simulink model "EZE557StEnCtrl"  (R2018b)
settings: Solver=FixedStepDiscrete  StartTime=0.0  StopTime=10.0  FixedStep=0.01  RelTol=1e-3
undefined symbols (not defined in the file or in its folder): data, KeSMSw4SSecRwLtStLgrstOtwdInwdClosePos1_Val, KeSMSw4SSecRwLtStLgrstUpwdDnwdClosePos1_Val, KeSMSw4SSecRwLtStLgrstUpwdDnwdClosePos2_Val, PassStBkReclnEn_Clear, PassStBkReclnEn_Set, PassStFwdBkwdEn_Clear, PassStFwdBkwdEn_Set, SecRwLtStBkReclnEn_Clear, SecRwLtStBkReclnEn_Set, SecRwLtStFwdBkwdEn_Clear, SecRwLtStFwdBkwdEn_Set, SecRwLtStLgrstInwdOtwdEn_Clear, SecRwLtStLgrstInwdOtwdEn_Set, SecRwLtStLgrstUpwdDnwdEn_Clear, SecRwLtStLgrstUpwdDnwdEn_Set, SecRwRtStBkReclnEn_Clear, SecRwRtStBkReclnEn_Set, SecRwRtStFwdBkwdEn_Clear, SecRwRtStFwdBkwdEn_Set, SecRwRtStLgrstInwdOtwdEn_Clear, SecRwRtStLgrstInwdOtwdEn_Set, SecRwRtStLgrstUpwdDnwdEn_Clear, SecRwRtStLgrstUpwdDnwdEn_Set, ThdRwLtStBkReclnEn_Clear, ThdRwLtStBkReclnEn_Set, ThdRwLtStCshnFldEn_Clear, ThdRwLtStCshnFldEn_Set, ThdRwLtStFwdBkwdEn_Clear, ThdRwLtStFwdBkwdEn_Set, ThdRwRtStBkReclnEn_Clear, ThdRwRtStBkReclnEn_Set, ThdRwRtStCshnFldEn_Clear, ThdRwRtStCshnFldEn_Set, ThdRwRtStFwdBkwdEn_Clear, ThdRwRtStFwdBkwdEn_Set, ZeroLEn_Clear, ZeroLEn_Set, ZeroREn_Clear, ZeroREn_Set
libraries: simulink x1
(part 2 of 2)

== system EZE557StEnCtrl/EZE557StEnCtrl_Cal_sys/Subsystem/If Action Subsystem24 ==
  Action Port : ActionPort
  Constant : Constant  Value=0  OutDataTypeStr=uint8
  ZeroREn_Set : FunctionCaller  FunctionPrototype=ZeroREn_Set(data)  InputArgumentSpecifications=uint8(1)  OutputArgumentSpecifications=<Enter example>
  wires:
  Constant/1 -> ZeroREn_Set/1

== system EZE557StEnCtrl/EZE557StEnCtrl_Cal_sys/Subsystem/If Action Subsystem25 ==
  note: Delete block
  Action Port : ActionPort
  Constant : Constant  Value=0  OutDataTypeStr=uint8
  SecRwLtStBkReclnEn_Set : FunctionCaller  FunctionPrototype=SecRwLtStBkReclnEn_Set(data)  InputArgumentSpecifications=uint8(1)  OutputArgumentSpecifications=<Enter example>
  wires:
  Constant/1 -> SecRwLtStBkReclnEn_Set/1

== system EZE557StEnCtrl/EZE557StEnCtrl_Cal_sys/Subsystem/If Action Subsystem26 ==
  note: Delete block
  Action Port : ActionPort
  Constant : Constant  Value=0  OutDataTypeStr=uint8
  SecRwRtStBkReclnEn_Set : FunctionCaller  FunctionPrototype=SecRwRtStBkReclnEn_Set(data)  InputArgumentSpecifications=uint8(1)  OutputArgumentSpecifications=<Enter example>
  wires:
  Constant/1 -> SecRwRtStBkReclnEn_Set/1

== system EZE557StEnCtrl/EZE557StEnCtrl_Cal_sys/Subsystem/If Action Subsystem27 ==
  note: Delete block
  Action Port : ActionPort
  Constant : Constant  Value=0  OutDataTypeStr=uint8
  PassStBkReclnEn_Clear : FunctionCaller  FunctionPrototype=PassStBkReclnEn_Clear(data)  InputArgumentSpecifications=uint8(1)
  wires:
  Constant/1 -> PassStBkReclnEn_Clear/1

== system EZE557StEnCtrl/EZE557StEnCtrl_Cal_sys/Subsystem/If Action Subsystem28 ==
  note: Delete block
  Action Port : ActionPort
  Constant : Constant  Value=0  OutDataTypeStr=uint8
  PassStBkReclnEn_Set : FunctionCaller  FunctionPrototype=PassStBkReclnEn_Set(data)  InputArgumentSpecifications=uint8(1)
  wires:
  Constant/1 -> PassStBkReclnEn_Set/1

== system EZE557StEnCtrl/EZE557StEnCtrl_Cal_sys/Subsystem/If Action Subsystem3 ==
  Action Port : ActionPort
  Constant : Constant  Value=0  OutDataTypeStr=uint8
  ThdRwLtStCshnFldEn_Set : FunctionCaller  FunctionPrototype=ThdRwLtStCshnFldEn_Set(data)  InputArgumentSpecifications=uint8(1)  OutputArgumentSpecifications=<Enter example>
  wires:
  Constant/1 -> ThdRwLtStCshnFldEn_Set/1

== system EZE557StEnCtrl/EZE557StEnCtrl_Cal_sys/Subsystem/If Action Subsystem4 ==
  Action Port : ActionPort
  Constant : Constant  Value=0  OutDataTypeStr=uint8
  ThdRwLtStCshnFldEn_Clear : FunctionCaller  FunctionPrototype=ThdRwLtStCshnFldEn_Clear(data)  InputArgumentSpecifications=uint8(1)  OutputArgumentSpecifications=<Enter example>
  wires:
  Constant/1 -> ThdRwLtStCshnFldEn_Clear/1

== system EZE557StEnCtrl/EZE557StEnCtrl_Cal_sys/Subsystem/If Action Subsystem5 ==
  Action Port : ActionPort
  Constant : Constant  Value=0  OutDataTypeStr=uint8
  ThdRwRtStCshnFldEn_Set : FunctionCaller  FunctionPrototype=ThdRwRtStCshnFldEn_Set(data)  InputArgumentSpecifications=uint8(1)  OutputArgumentSpecifications=<Enter example>
  wires:
  Constant/1 -> ThdRwRtStCshnFldEn_Set/1

== system EZE557StEnCtrl/EZE557StEnCtrl_Cal_sys/Subsystem/If Action Subsystem6 ==
  Action Port : ActionPort
  Constant : Constant  Value=0  OutDataTypeStr=uint8
  ThdRwRtStCshnFldEn_Clear : FunctionCaller  FunctionPrototype=ThdRwRtStCshnFldEn_Clear(data)  InputArgumentSpecifications=uint8(1)  OutputArgumentSpecifications=<Enter example>
  wires:
  Constant/1 -> ThdRwRtStCshnFldEn_Clear/1

== system EZE557StEnCtrl/EZE557StEnCtrl_Cal_sys/Subsystem/If Action Subsystem7 ==
  note: Delete block
  Action Port : ActionPort
  Constant : Constant  Value=0  OutDataTypeStr=uint8
  PassStFwdBkwdEn_Clear : FunctionCaller  FunctionPrototype=PassStFwdBkwdEn_Clear(data)  InputArgumentSpecifications=uint8(1)
  wires:
  Constant/1 -> PassStFwdBkwdEn_Clear/1

== system EZE557StEnCtrl/EZE557StEnCtrl_Cal_sys/Subsystem/If Action Subsystem8 ==
  note: Delete block
  Action Port : ActionPort
  Constant : Constant  Value=0  OutDataTypeStr=uint8
  PassStFwdBkwdEn_Set : FunctionCaller  FunctionPrototype=PassStFwdBkwdEn_Set(data)  InputArgumentSpecifications=uint8(1)
  wires:
  Constant/1 -> PassStFwdBkwdEn_Set/1

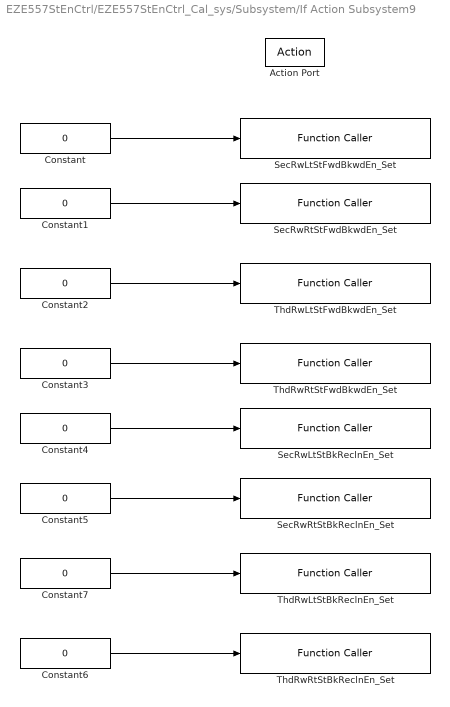
== system EZE557StEnCtrl/EZE557StEnCtrl_Cal_sys/Subsystem/If Action Subsystem9 ==
  Action Port : ActionPort
  Constant{,1..7} (8 alike) : Constant  Value=0  OutDataTypeStr=uint8
  SecRwLtStBkReclnEn_Set : FunctionCaller  FunctionPrototype=SecRwLtStBkReclnEn_Set(data)  InputArgumentSpecifications=uint8(1)  OutputArgumentSpecifications=<Enter example>
  SecRwLtStFwdBkwdEn_Set : FunctionCaller  FunctionPrototype=SecRwLtStFwdBkwdEn_Set(data)  InputArgumentSpecifications=uint8(1)  OutputArgumentSpecifications=<Enter example>
  SecRwRtStBkReclnEn_Set : FunctionCaller  FunctionPrototype=SecRwRtStBkReclnEn_Set(data)  InputArgumentSpecifications=uint8(1)  OutputArgumentSpecifications=<Enter example>
  SecRwRtStFwdBkwdEn_Set : FunctionCaller  FunctionPrototype=SecRwRtStFwdBkwdEn_Set(data)  InputArgumentSpecifications=uint8(1)  OutputArgumentSpecifications=<Enter example>
  ThdRwLtStBkReclnEn_Set : FunctionCaller  FunctionPrototype=ThdRwLtStBkReclnEn_Set(data)  InputArgumentSpecifications=uint8(1)  OutputArgumentSpecifications=<Enter example>
  ThdRwLtStFwdBkwdEn_Set : FunctionCaller  FunctionPrototype=ThdRwLtStFwdBkwdEn_Set(data)  InputArgumentSpecifications=uint8(1)  OutputArgumentSpecifications=<Enter example>
  ThdRwRtStBkReclnEn_Set : FunctionCaller  FunctionPrototype=ThdRwRtStBkReclnEn_Set(data)  InputArgumentSpecifications=uint8(1)  OutputArgumentSpecifications=<Enter example>
  ThdRwRtStFwdBkwdEn_Set : FunctionCaller  FunctionPrototype=ThdRwRtStFwdBkwdEn_Set(data)  InputArgumentSpecifications=uint8(1)  OutputArgumentSpecifications=<Enter example>
  wires:
  Constant/1 -> SecRwLtStFwdBkwdEn_Set/1
  Constant1/1 -> SecRwRtStFwdBkwdEn_Set/1
  Constant2/1 -> ThdRwLtStFwdBkwdEn_Set/1
  Constant3/1 -> ThdRwRtStFwdBkwdEn_Set/1
  Constant4/1 -> SecRwLtStBkReclnEn_Set/1
  Constant5/1 -> SecRwRtStBkReclnEn_Set/1
  Constant6/1 -> ThdRwRtStBkReclnEn_Set/1
  Constant7/1 -> ThdRwLtStBkReclnEn_Set/1

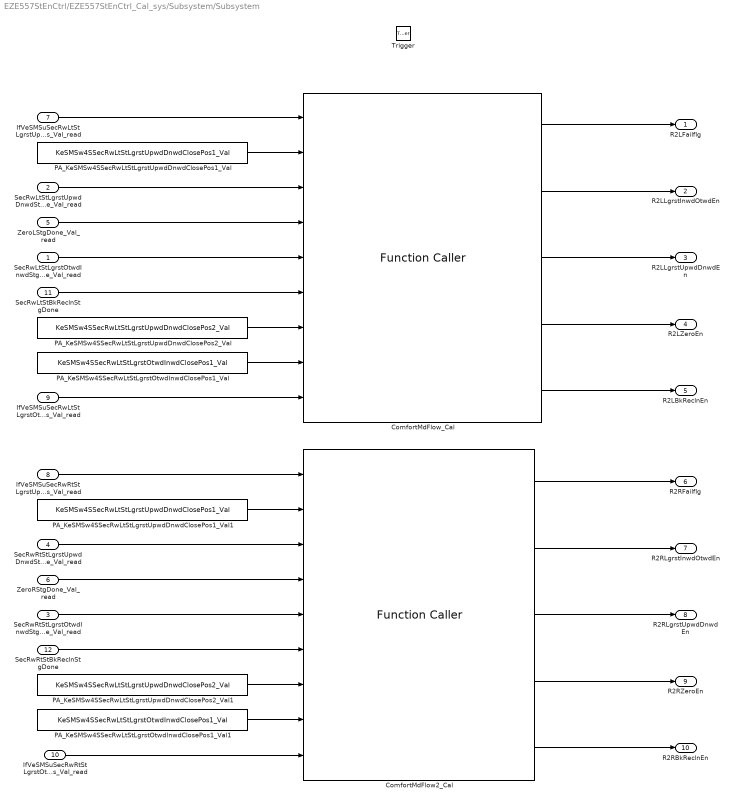
== system EZE557StEnCtrl/EZE557StEnCtrl_Cal_sys/Subsystem/Subsystem ==
  SecRwLtStLgrstOtwdInwdStgDone_Val_read : Inport
  SecRwLtStLgrstUpwdDnwdStgDone_Val_read : Inport  Port=2
  SecRwRtStLgrstOtwdInwdStgDone_Val_read : Inport  Port=3
  SecRwRtStLgrstUpwdDnwdStgDone_Val_read : Inport  Port=4
  ZeroLStgDone_Val_read : Inport  Port=5
  ZeroRStgDone_Val_read : Inport  Port=6
  IfVeSMSuSecRwLtStLgrstUpwdDnwdPos_Val_read : Inport  Port=7
  IfVeSMSuSecRwRtStLgrstUpwdDnwdPos_Val_read : Inport  Port=8
  IfVeSMSuSecRwLtStLgrstOtwdInwdPos_Val_read : Inport  Port=9
  IfVeSMSuSecRwRtStLgrstOtwdInwdPos_Val_read : Inport  Port=10
  SecRwLtStBkReclnStgDone : Inport  Port=11
  SecRwRtStBkReclnStgDone : Inport  Port=12
  Trigger : TriggerPort  TriggerType=function-call  VariantControl=Variant  PortDimensions=1
  ComfortMdFlow2_Cal : FunctionCaller  FunctionPrototype=[Failflg,LgrstInwdOtwdEn,LgrstUpwdDnwdEn,ZeroEn,BkReclnEn] = ComfortMdFlow2_Cal(LgrstUpwdDnwdPos,LgrstUpwdDnwdClosePos1,LgrstUpwdStgDone,ZeroStgDone,LgrstInwdStgDone,BkReclnStgDone,LgrstUpwdDnwdClosePos2,LgrstInwdOtwdClosePos1,LgrstInwdOtwdPos)  InputArgumentSpecifications=uint16(1), uint16(1), boolean(true), boolean(true), boolean(true), boolean(true), uint16(1), uint16(1), uint16(1)  OutputArgumentSpecifications=boolean(true), boolean(true), boolean(true), boolean(true), boolean(true)
  ComfortMdFlow_Cal : FunctionCaller  FunctionPrototype=[Failflg,LgrstInwdOtwdEn,LgrstUpwdDnwdEn,ZeroEn,BkReclnEn] = ComfortMdFlow_Cal(LgrstUpwdDnwdPos,LgrstUpwdDnwdClosePos1,LgrstUpwdStgDone,ZeroStgDone,LgrstInwdStgDone,BkReclnStgDone,LgrstUpwdDnwdClosePos2,LgrstInwdOtwdClosePos1,LgrstInwdOtwdPos)  InputArgumentSpecifications=uint16(1), uint16(1), boolean(true), boolean(true), boolean(true), boolean(true), uint16(1), uint16(1), uint16(1)  OutputArgumentSpecifications=boolean(true), boolean(true), boolean(true), boolean(true), boolean(true)
  PA_KeSMSw4SSecRwLtStLgrstOtwdInwdClosePos1_Val : Constant  Value=KeSMSw4SSecRwLtStLgrstOtwdInwdClosePos1_Val
  PA_KeSMSw4SSecRwLtStLgrstOtwdInwdClosePos1_Val1 : Constant  Value=KeSMSw4SSecRwLtStLgrstOtwdInwdClosePos1_Val
  PA_KeSMSw4SSecRwLtStLgrstUpwdDnwdClosePos1_Val : Constant  Value=KeSMSw4SSecRwLtStLgrstUpwdDnwdClosePos1_Val
  PA_KeSMSw4SSecRwLtStLgrstUpwdDnwdClosePos1_Val1 : Constant  Value=KeSMSw4SSecRwLtStLgrstUpwdDnwdClosePos1_Val
  PA_KeSMSw4SSecRwLtStLgrstUpwdDnwdClosePos2_Val : Constant  Value=KeSMSw4SSecRwLtStLgrstUpwdDnwdClosePos2_Val
  PA_KeSMSw4SSecRwLtStLgrstUpwdDnwdClosePos2_Val1 : Constant  Value=KeSMSw4SSecRwLtStLgrstUpwdDnwdClosePos2_Val
  R2LFailflg : Outport  VectorParamsAs1DForOutWhenUnconnected=off
  R2LLgrstInwdOtwdEn : Outport  Port=2  VectorParamsAs1DForOutWhenUnconnected=off
  R2LLgrstUpwdDnwdEn : Outport  Port=3  VectorParamsAs1DForOutWhenUnconnected=off
  R2LZeroEn : Outport  Port=4  VectorParamsAs1DForOutWhenUnconnected=off
  R2LBkReclnEn : Outport  Port=5  VectorParamsAs1DForOutWhenUnconnected=off
  R2RFailflg : Outport  Port=6  VectorParamsAs1DForOutWhenUnconnected=off
  R2RLgrstInwdOtwdEn : Outport  Port=7  VectorParamsAs1DForOutWhenUnconnected=off
  R2RLgrstUpwdDnwdEn : Outport  Port=8  VectorParamsAs1DForOutWhenUnconnected=off
  R2RZeroEn : Outport  Port=9  VectorParamsAs1DForOutWhenUnconnected=off
  R2RBkReclnEn : Outport  Port=10  VectorParamsAs1DForOutWhenUnconnected=off
  wires:
  SecRwRtStLgrstUpwdDnwdStgDone_Val_read/1 -> ComfortMdFlow2_Cal/3
  SecRwRtStLgrstOtwdInwdStgDone_Val_read/1 -> ComfortMdFlow2_Cal/5
  IfVeSMSuSecRwRtStLgrstUpwdDnwdPos_Val_read/1 -> ComfortMdFlow2_Cal/1
  ComfortMdFlow_Cal/1 -> R2LFailflg/1
  ZeroRStgDone_Val_read/1 -> ComfortMdFlow2_Cal/4
  SecRwLtStLgrstOtwdInwdStgDone_Val_read/1 -> ComfortMdFlow_Cal/5
  SecRwLtStLgrstUpwdDnwdStgDone_Val_read/1 -> ComfortMdFlow_Cal/3
  ZeroLStgDone_Val_read/1 -> ComfortMdFlow_Cal/4
  IfVeSMSuSecRwLtStLgrstUpwdDnwdPos_Val_read/1 -> ComfortMdFlow_Cal/1
  SecRwLtStBkReclnStgDone/1 -> ComfortMdFlow_Cal/6
  SecRwRtStBkReclnStgDone/1 -> ComfortMdFlow2_Cal/6
  ComfortMdFlow_Cal/2 -> R2LLgrstInwdOtwdEn/1
  ComfortMdFlow_Cal/3 -> R2LLgrstUpwdDnwdEn/1
  ComfortMdFlow_Cal/4 -> R2LZeroEn/1
  ComfortMdFlow_Cal/5 -> R2LBkReclnEn/1
  ComfortMdFlow2_Cal/5 -> R2RBkReclnEn/1
  ComfortMdFlow2_Cal/4 -> R2RZeroEn/1
  ComfortMdFlow2_Cal/3 -> R2RLgrstUpwdDnwdEn/1
  ComfortMdFlow2_Cal/2 -> R2RLgrstInwdOtwdEn/1
  ComfortMdFlow2_Cal/1 -> R2RFailflg/1
  PA_KeSMSw4SSecRwLtStLgrstUpwdDnwdClosePos2_Val1/1 -> ComfortMdFlow2_Cal/7
  IfVeSMSuSecRwRtStLgrstOtwdInwdPos_Val_read/1 -> ComfortMdFlow2_Cal/9
  PA_KeSMSw4SSecRwLtStLgrstUpwdDnwdClosePos2_Val/1 -> ComfortMdFlow_Cal/7
  IfVeSMSuSecRwLtStLgrstOtwdInwdPos_Val_read/1 -> ComfortMdFlow_Cal/9
  PA_KeSMSw4SSecRwLtStLgrstOtwdInwdClosePos1_Val/1 -> ComfortMdFlow_Cal/8
  PA_KeSMSw4SSecRwLtStLgrstUpwdDnwdClosePos1_Val/1 -> ComfortMdFlow_Cal/2
  PA_KeSMSw4SSecRwLtStLgrstUpwdDnwdClosePos1_Val1/1 -> ComfortMdFlow2_Cal/2
  PA_KeSMSw4SSecRwLtStLgrstOtwdInwdClosePos1_Val1/1 -> ComfortMdFlow2_Cal/8

== system EZE557StEnCtrl/EZE557StEnCtrl_Cal_sys/Subsystem/Subsystem1 ==
  Enable : EnablePort
  Constant3 : Constant  Value=0  OutDataTypeStr=uint8
  SecRwLtStBkReclnEn_Clear : FunctionCaller  FunctionPrototype=SecRwLtStBkReclnEn_Clear(data)  InputArgumentSpecifications=uint8(1)  OutputArgumentSpecifications=<Enter example>
  wires:
  Constant3/1 -> SecRwLtStBkReclnEn_Clear/1

== system EZE557StEnCtrl/EZE557StEnCtrl_Cal_sys/Subsystem/Subsystem2 ==
  Enable : EnablePort
  Constant4 : Constant  Value=0  OutDataTypeStr=uint8
  SecRwRtStBkReclnEn_Clear : FunctionCaller  FunctionPrototype=SecRwRtStBkReclnEn_Clear(data)  InputArgumentSpecifications=uint8(1)  OutputArgumentSpecifications=<Enter example>
  wires:
  Constant4/1 -> SecRwRtStBkReclnEn_Clear/1

== stateflow chart EZE557StEnCtrl/EZE557StEnCtrl_Cal_sys/Subsystem/Chart ==
  (default) -> (junction 223) : {
      | R2LBkReclinFirstStepPassFlg=0;
      | R2RBkReclinFirstStepPassFlg=0;
      | R3LBkReclnEn =0;
      | R3RBkReclnEn =0;
      | R3LCshnFldEn = 0;
      | R3RCshnFldEn = 0;
      | Stage2En = 0;
      | PassStFwdBkwdEn=0;
      | PassStBkReclnEn=0;
      | }
  (junction 223) -> (junction 222) [order 1] : [!PassStFwdBkwdStgDone]
  (junction 223) -> (junction 227) [order 2]
  (junction 222) -> (junction 226) : {PassStFwdBkwdEn=1;}
  (junction 226) -> (junction 227)
  (junction 227) -> (junction 228)
  (junction 228) -> (junction 229) [order 1] : [!PassStBkReclnStgDone]
  (junction 228) -> (junction 231) [order 2]
  (junction 229) -> (junction 230) : {PassStBkReclnEn=1;}
  (junction 230) -> (junction 231)
  (junction 231) -> (junction 1)
  (junction 1) -> (junction 3) [order 1] : [(IfVeSMSuThdRwLtStCshnFldUpwdDnwdPos>=4000)]
  (junction 3) -> (junction 208) [order 1] : [(IfVeSMSuThdRwRtStCshnFldUpwdDnwdPos>=4000)]
  (junction 1) -> (junction 9) [order 2]
  (junction 3) -> (junction 7) [order 2] : {
      | R2LBkReclinFirstStepPassFlg=1;
      | }
  (junction 208) -> (junction 210) : {
      | R2RBkReclinFirstStepPassFlg=1;
      | }
  (junction 7) -> (junction 9)
  (junction 210) -> (junction 7)
  (junction 9) -> (junction 75)
  (junction 75) -> (junction 77) [order 1] : [IfVeSMSuSecRwLtStBkReclnUpwdDnwdPos<=EZER2LBkReclnUpwdDnwdTrgtPos1]
  (junction 75) -> (junction 81) [order 2]
  (junction 77) -> (junction 79) : {
      | R2LBkReclinFirstStepPassFlg=1;
      | }
  (junction 79) -> (junction 81)
  (junction 81) -> (junction 84)
  (junction 84) -> (junction 86) [order 1] : [IfVeSMSuSecRwRtStBkReclnUpwdDnwdPos<=EZER2RBkReclnUpwdDnwdTrgtPos1]
  (junction 84) -> (junction 90) [order 2]
  (junction 86) -> (junction 88) : {
      | R2RBkReclinFirstStepPassFlg=1;
      | }
  (junction 88) -> (junction 90)
  (junction 90) -> (junction 95)
  (junction 95) -> (junction 97) [order 1] : [!Stage1Done]
  (junction 95) -> (junction 101) [order 2]
  (junction 97) -> (junction 118) : {
      | TrigComfortMd;
      | }
  (junction 118) -> (junction 119) [order 1] : [IfVeSMSuThdRwRtStCshnFldUpwdDnwdPos>=4000]
  (junction 119) -> (junction 121) [order 1] : [!FirstStgR3RBkReclnNotMovFlg && !ThdRwRtStBkReclnStgDone]
  (junction 118) -> (junction 131) [order 2]
  (junction 119) -> (junction 128) [order 2]
  (junction 121) -> (junction 123) : {
      | R3RBkReclnEn =1;
      | }
  (junction 131) -> (junction 133) [order 1] : [IfVeSMSuSecRwRtStBkReclnUpwdDnwdPos<=(EZER2RBkReclnUpwdDnwdTrgtPos1)]
  (junction 131) -> (junction 141) [order 2]
  (junction 133) -> (junction 135)
  (junction 141) -> (junction 135) [order 1] : [SecRwRtStBkReclnStgDone]
  (junction 135) -> (junction 182) [order 1] : [ThdRwRtStCshnFldStgDone]
  (junction 141) -> (junction 137) [order 2]
  (junction 135) -> (junction 148) [order 2] : {
      | R3RCshnFldEn =1;
      | }
  (junction 182) -> (junction 184)
  (junction 148) -> (junction 137)
  (junction 184) -> (junction 148)
  (junction 137) -> (junction 150)
  (junction 128) -> (junction 150)
  (junction 123) -> (junction 128)
  (junction 150) -> (junction 153)
  (junction 153) -> (junction 155) [order 1] : [IfVeSMSuThdRwLtStCshnFldUpwdDnwdPos>=4000]
  (junction 155) -> (junction 157) [order 1] : [!FirstStgR3LBkReclnNotMovFlg &&!ThdRwLtStBkReclnStgDone]
  (junction 153) -> (junction 161) [order 2]
  (junction 155) -> (junction 177) [order 2]
  (junction 157) -> (junction 159) : {
      | R3LBkReclnEn =1;
      | }
  (junction 161) -> (junction 163) [order 1] : [IfVeSMSuSecRwLtStBkReclnUpwdDnwdPos<=(EZER2LBkReclnUpwdDnwdTrgtPos1)&&...
      | IfVeSMSuSecRwRtStBkReclnUpwdDnwdPos<=(EZER2RBkReclnUpwdDnwdTrgtPos1)]
  (junction 161) -> (junction 167) [order 2]
  (junction 163) -> (junction 165)
  (junction 167) -> (junction 165) [order 1] : [ SecRwLtStBkReclnStgDone&&SecRwRtStBkReclnStgDone]
  (junction 165) -> (junction 187) [order 1] : [ThdRwLtStCshnFldStgDone]
  (junction 167) -> (junction 173) [order 2]
  (junction 165) -> (junction 171) [order 2] : {
      | R3LCshnFldEn =1;
      | }
  (junction 187) -> (junction 189)
  (junction 101) -> (junction 104) [order 1] : [!Stage2Done]
  (junction 101) -> (junction 109) [order 2]
  (junction 104) -> (junction 106) : {Stage2En = 1;}
  (junction 106) -> (junction 109)
  (junction 173) -> (junction 106)
  (junction 171) -> (junction 173)
  (junction 189) -> (junction 171)
  (junction 177) -> (junction 189)
  (junction 159) -> (junction 177)
  (junction 109) -> (junction 196)
  data: PassStBkReclnStgDone input; PassStFwdBkwdStgDone input; ThdRwLtStBkReclnStgDone input; ThdRwRtStBkReclnStgDone input; IfVeSMSuThdRwLtStCshnFldUpwdDnwdPos input; IfVeSMSuThdRwRtStCshnFldUpwdDnwdPos input; IfVeSMSuSecRwLtStBkReclnUpwdDnwdPos input; IfVeSMSuSecRwRtStBkReclnUpwdDnwdPos input; EZER2LBkReclnUpwdDnwdTrgtPos1 input; EZER2RBkReclnUpwdDnwdTrgtPos1 input; R2LBkReclinFirstStepPassFlg output boolean; R2RBkReclinFirstStepPassFlg output boolean; Stage1Done input boolean; Stage2Done input boolean; FirstStgR3LBkReclnNotMovFlg input boolean; FirstStgR3RBkReclnNotMovFlg input boolean; R3RBkReclnEn output boolean; R3LCshnFldEn output boolean; R3RCshnFldEn output boolean; Stage2En output boolean; ThdRwRtStCshnFldStgDone input; ThdRwLtStCshnFldStgDone input; SecRwRtStBkReclnStgDone input; SecRwLtStBkReclnStgDone input; R3LBkReclnEn output boolean; PassStFwdBkwdEn output boolean; PassStBkReclnEn output boolean; R3LCshnFldEn2 output boolean; R3LCshnFldEn3 output boolean
  events: TrigComfortMd output FUNCTION_CALL_EVENT
